simulink model "AM_envelope2_2023b"  (R2023b)
settings: Solver=ode45  StartTime=0.0  StopTime=10  RelTol=1e-3  EnableMultiTasking=on
values from neighbouring files (symbols this model uses):
  seed = input('Enter your student ID: ')    [DSBAMsignals.m]    (also in DSBAMsignals_rand.m; DSB_SC_sinusoidals.m)
libraries: dspfdesign x2
settings Model: Creator=morelos_zaragoza  LastModifiedBy=14083
settings SolverCC: AlgebraicLoopSolver=TrustRegion
settings DataIOCC: LimitDataPoints=on  SaveFormat=Array  SignalLoggingSaveFormat=ModelDataLogs  ReturnWorkspaceOutputs=off
settings OptimizationCC: ExpressionDepthLimit=2147483647  InitFltsAndDblsToZero=on  LifeSpan=inf
settings DebuggingCC: SaveWithParameterizedLinksMsg=none  UnderspecifiedInitializationDetection=Classic  MergeDetectMultiDrivingBlocksExec=none  SignalResolutionControl=TryResolveAllWithWarning  SolverPrmCheckMsg=warning  MultiTaskDSMMsg=warning  MultiTaskCondExecSysMsg=none  FcnCallInpInsideContextMsg=warning  UnconnectedInputMsg=warning  UnconnectedOutputMsg=warning  UnconnectedLineMsg=warning  StateNameClashWarn=warning  SFUnexpectedBacktrackingDiag=warning  SFNoUnconditionalDefaultTransitionDiag=warning  SFExecutionAtInitializationDiag=none  ArithmeticOperatorsInVariantConditions=warning
settings HardwareCC: ProdBitPerPointer=32  ProdBitPerSizeT=32  ProdBitPerPtrDiffT=32  ProdLargestAtomicFloat=None  ProdIntDivRoundTo=Undefined  ProdEndianess=Unspecified  ProdWordSize=32  ProdHWDeviceType=32-bit Generic
settings ModelReferenceCC: EnableRefExpFcnMdlSchedulingChecks=on  PropagateSignalLabelsOutOfModel=off
settings SFSimCC: SimUseLocalCustomCode=off  CustomCodeUndefinedFunction=UseInterfaceOnly
settings RTWCC: RTWUseLocalCustomCode=off
settings CodeAppCC: StateflowObjectComments=on
settings GRTTargetCC: TargetFcnLib=ansi_tfl_tmw.mat  TargetLangStandard=C89/C90 (ANSI)  CombineOutputUpdateFcns=off  GRTInterface=on
settings ConfigComp: CovMetricSettings=dw  CovSaveCumulativeToWorkspaceVar=on  CovSaveSingleToWorkspaceVar=on  CovExternalEMLEnable=off

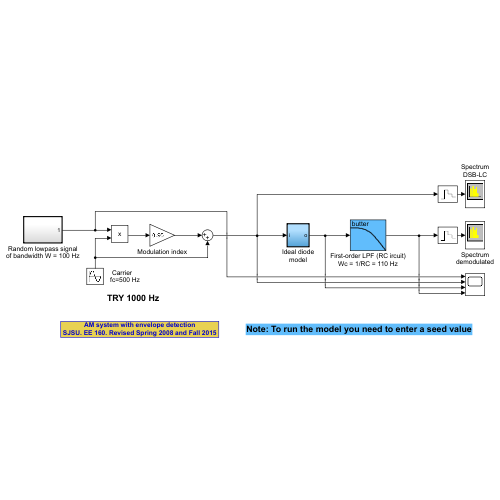
[thumbnail: Simulink's stored preview of the top-level diagram]
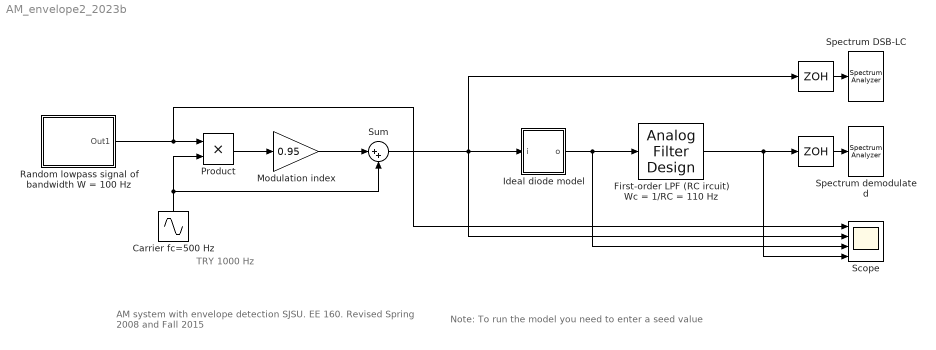
== system AM_envelope2_2023b ==
  note: TRY 1000 Hz
  note: AM system with envelope detection
      | SJSU. EE 160. Revised Spring 2008 and Fall 2015
  note: Note: To run the model you need to enter a seed value
  "  " : ZeroOrderHold  SampleTime=1/(25*90)
  "   " : ZeroOrderHold  SampleTime=1/(25*90)
  "   Carrier fc=500 Hz" : Sin  Frequency=2*pi*500  SampleTime=0
  First-order LPF (RC ircuit) Wc = 1/RC = 110 Hz : dspfdesign/Analog Filter Design  method=Butterworth  filttype=Lowpass  N=1  Wlo=2*pi*110  Whi=2*pi*110  Rp=2  Rs=60
  Ideal diode model : Subsystem  TreatAsAtomicUnit=on
  Modulation index : Gain  Gain=0.95
  Product : Product  RndMeth=Zero
  Random lowpass signal of bandwidth W = 100 Hz : Subsystem  TreatAsAtomicUnit=on
  Scope : Scope  NumInputPorts=4
  Spectrum DSB-LC : SpectrumAnalyzer  WindowPosition=[777.000000,402.000000,588.000000,281.000000,]  Visible=on  ScopeFrameLocation=window  Method=Welch  SampleRate=2250  AxesScaling=Manual  Span=2250  StartFrequency=-1125  StopFrequency=1125  FrequencyResolutionMethod=Window length  FFTLengthSource=Property  FFTLength=512  WindowLength=512  OverlapPercent=25  AveragingMethod=Running  SpectralAverages=10  YLabel=Magnitude  YLimits=[-60,25]  DefaultConfigurationName=spbscopes.SpectrumAnalyzerBlockCfg  IsFrequencyInputMode=0  FrequencyVectorPort=0  FrequencyVectorFromPort=0  FrequencyInputRBWPort=0  FrequencyInputRBWFromPort=0  SegLen=512
  Spectrum demodulated : SpectrumAnalyzer  WindowPosition=[775.000000,45.000000,589.000000,272.000000,]  Visible=on  ScopeFrameLocation=window  Method=Welch  SampleRate=2250  AxesScaling=Manual  Span=2250  StartFrequency=-1125  StopFrequency=1125  FrequencyResolutionMethod=Window length  FFTLengthSource=Property  FFTLength=512  WindowLength=512  OverlapPercent=25  AveragingMethod=Running  SpectralAverages=10  YLabel=Magnitude  YLimits=[-60,25]  DefaultConfigurationName=spbscopes.SpectrumAnalyzerBlockCfg  IsFrequencyInputMode=0  FrequencyVectorPort=0  FrequencyVectorFromPort=0  FrequencyInputRBWPort=0  FrequencyInputRBWFromPort=0  SegLen=512
  Sum : Sum  Inputs=|++
  wires:
  Random lowpass signal of bandwidth W = 100 Hz/1(Out1) -> Product/1, Scope/1
  "   Carrier fc=500 Hz"/1 -> Product/2, Sum/2
  "  "/1 -> Spectrum DSB-LC/1
  "   "/1 -> Spectrum demodulated/1
  First-order LPF (RC ircuit) Wc = 1/RC = 110 Hz/1 -> "   "/1, Scope/4
  Ideal diode model/1(o) -> First-order LPF (RC ircuit) Wc = 1/RC = 110 Hz/1, Scope/3
  Modulation index/1 -> Sum/1
  Product/1 -> Modulation index/1
  Sum/1 -> Ideal diode model/1(i), "  "/1, Scope/2

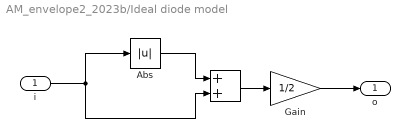
== system AM_envelope2_2023b/Ideal diode model ==
  i : Inport
  " " : Sum
  Abs : Abs  SaturateOnIntegerOverflow=off
  Gain : Gain  Gain=1/2
  o : Outport
  wires:
  i/1 -> Abs/1, " "/2
  Abs/1 -> " "/1
  " "/1 -> Gain/1
  Gain/1 -> o/1

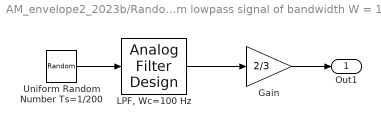
== system AM_envelope2_2023b/Random lowpass signal of bandwidth W = 100 Hz ==
  Gain : Gain  Gain=2/3
  "LPF, Wc=100 Hz" : dspfdesign/Analog Filter Design  method=Butterworth  filttype=Lowpass  N=18  Wlo=2*pi*100  Whi=2*pi*110  Rp=2  Rs=40
  Uniform Random Number Ts=1/200 : UniformRandomNumber  Seed=seed  SampleTime=1/200
  Out1 : Outport
  wires:
  Uniform Random Number Ts=1/200/1 -> "LPF, Wc=100 Hz"/1
  "LPF, Wc=100 Hz"/1 -> Gain/1
  Gain/1 -> Out1/1
